simulink model "drone_nao_linear_V3_MF_LQR"  (R2015a)
settings: Solver=ode45  StartTime=0.0  StopTime=30  FixedStep=.001  RelTol=1e-3
values from neighbouring files (symbols this model uses):
  Cx = 1.33    [projeto_Drone_LQR_pratico.m]
  Cy = 1.95    [projeto_Drone_LQR_pratico.m]
  d_fi = 1.35    [projeto_Drone_LQR_pratico.m]
  d_teta = 0.99    [projeto_Drone_LQR_pratico.m]
  Fi_max = 0.4171/2    (= 0.20855)    [projeto_Drone_LQR_pratico.m]
  g = 0.165/(pi/180)    (= 9.45380361966)    [projeto_Drone_LQR_pratico.m]
  K_psi_p = 1    [projeto_Drone_LQR_pratico.m]
  K_z_p = 1    [projeto_Drone_LQR_pratico.m]
  Kipsi = -Ka_psi(1,3)    [projeto_Drone_LQR_pratico.m]
  Kix = -Ka_x(1,5)    [projeto_Drone_LQR_pratico.m]
  Kiy = -Ka_y(1,5)    [projeto_Drone_LQR_pratico.m]
  Kiz = -Ka_z(1,3)    [projeto_Drone_LQR_pratico.m]
  Kpsi = -Ka_psi(1,1:2)    [projeto_Drone_LQR_pratico.m]
  Kx = -Ka_x(1,1:4)    [projeto_Drone_LQR_pratico.m]
  Ky = -Ka_y(1,1:4)    [projeto_Drone_LQR_pratico.m]
  Kz = -Ka_z(1,1:2)    [projeto_Drone_LQR_pratico.m]
  omega_fi = 14.43    [projeto_Drone_LQR_pratico.m]
  omega_teta = 13.14    [projeto_Drone_LQR_pratico.m]
  Psi_p_max = 92.75*(pi/180)    (= 1.61879288122)    [projeto_Drone_LQR_pratico.m]
  T = 5    [projeto_Drone_LQR_pratico.m]
  Tau_psi_p = 0.51    [projeto_Drone_LQR_pratico.m]
  Tau_z_p = 0.88    [projeto_Drone_LQR_pratico.m]
  Teta_max = 0.4184/2    (= 0.2092)    [projeto_Drone_LQR_pratico.m]
  z_p_max = 1.35    [projeto_Drone_LQR_pratico.m]
libraries: simulink_extras x3
settings Model: Creator=Humberto  LastModifiedBy=Humberto

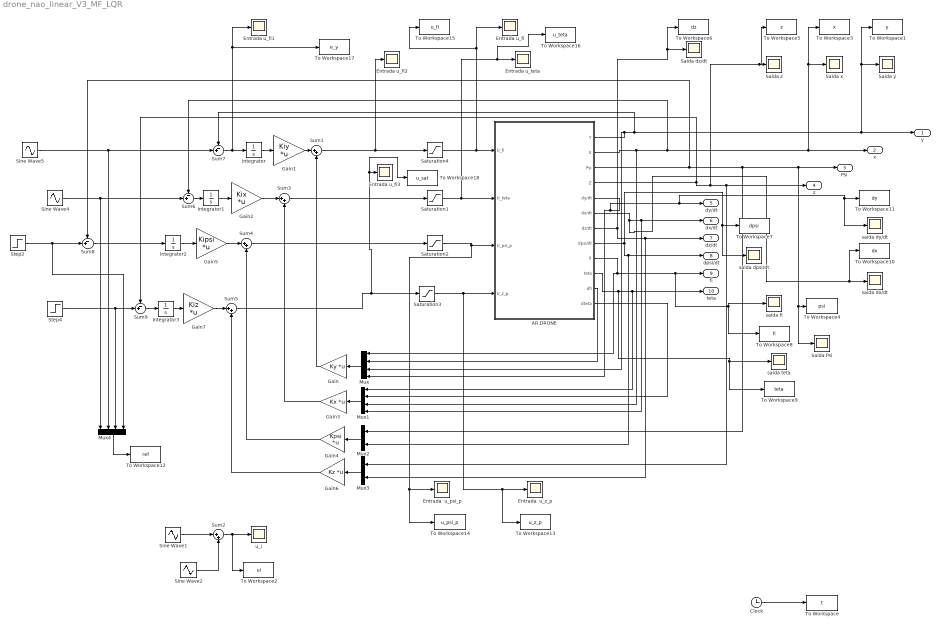
== system drone_nao_linear_V3_MF_LQR ==
  AR.DRONE : Subsystem
      mask Display: color('blue');port_label('output',1,'x')
  Clock : Clock
  Entrada  u_psi_p : Scope
      settings: SaveName=ScopeData17
  Entrada  u_z_p : Scope
      settings: SaveName=ScopeData16
  Entrada u_fi{,1..3} (4 alike) : Scope
      Entrada u_fi settings: SaveName=ScopeData14
      Entrada u_fi1 settings: SaveName=ScopeData22
      Entrada u_fi2 settings: SaveName=ScopeData23
      Entrada u_fi3 settings: SaveName=ScopeData24
  Entrada u_teta : Scope
      settings: SaveName=ScopeData15
  Gain : Gain  Gain=Ky  Multiplication=Matrix(K*u)
  Gain1 : Gain  Gain=Kiy  Multiplication=Matrix(K*u)
  Gain2 : Gain  Gain=Kix  Multiplication=Matrix(K*u)
  Gain3 : Gain  Gain=Kx  Multiplication=Matrix(K*u)
  Gain4 : Gain  Gain=Kpsi  Multiplication=Matrix(K*u)
  Gain5 : Gain  Gain=Kipsi  Multiplication=Matrix(K*u)
  Gain6 : Gain  Gain=Kz  Multiplication=Matrix(K*u)
  Gain7 : Gain  Gain=Kiz  Multiplication=Matrix(K*u)
  Integrator{,1..3} (4 alike) : Integrator
  Mux : Mux
  Mux1 : Mux
  Mux2 : Mux  Inputs=2
  Mux3 : Mux  Inputs=2
  Mux4 : Mux
  Saida Psi : Scope
      settings: SaveName=ScopeData2
  Saida dz/dt : Scope
      settings: SaveName=ScopeData19
  Saida x : Scope
  Saida y : Scope
  Saida z : Scope
      settings: SaveName=ScopeData3
  Saturation{1..4} (4 alike) : Saturate  UpperLimit=1  LowerLimit=-1
  Sine Wave1 : Sin  Amplitude=0.5  Frequency=2*pi/T  SampleTime=0
  Sine Wave2 : Sin  Amplitude=0.3  Frequency=2*pi/(0.2*T)  SampleTime=0
  Sine Wave4 : Sin  Frequency=0.8  SampleTime=0
  Sine Wave5 : Sin  Frequency=0.8  Phase=pi/2  SampleTime=0
  Step2 : Step  Time=0  After=0  SampleTime=0
  Step4 : Step  Time=0  After=1.2  SampleTime=0
  Sum{1..5} (5 alike) : Sum  Inputs=|++
  Sum{6..9} (4 alike) : Sum  Inputs=-+|
  To Workspace : ToWorkspace  VariableName=t  SampleTime=-1
  To Workspace1 : ToWorkspace  VariableName=y  SampleTime=-1
  To Workspace10 : ToWorkspace  VariableName=dx  SampleTime=-1
  To Workspace11 : ToWorkspace  VariableName=dy  SampleTime=-1
  To Workspace12 : ToWorkspace  VariableName=ref  SampleTime=-1
  To Workspace13 : ToWorkspace  VariableName=u_z_p  SampleTime=-1
  To Workspace14 : ToWorkspace  VariableName=u_psi_p  SampleTime=-1
  To Workspace15 : ToWorkspace  VariableName=u_fi  SampleTime=-1
  To Workspace16 : ToWorkspace  VariableName=u_teta  SampleTime=-1
  To Workspace17 : ToWorkspace  VariableName=e_y  SampleTime=-1
  To Workspace18 : ToWorkspace  VariableName=u_sat  SampleTime=-1
  To Workspace2 : ToWorkspace  VariableName=ui  SampleTime=-1
  To Workspace3 : ToWorkspace  VariableName=x  SampleTime=-1
  To Workspace4 : ToWorkspace  VariableName=psi  SampleTime=-1
  To Workspace5 : ToWorkspace  VariableName=z  SampleTime=-1
  To Workspace6 : ToWorkspace  VariableName=dz  SampleTime=-1
  To Workspace7 : ToWorkspace  VariableName=dpsi  SampleTime=-1
  To Workspace8 : ToWorkspace  VariableName=fi  SampleTime=-1
  To Workspace9 : ToWorkspace  VariableName=teta  SampleTime=-1
  saida dpsi/dt : Scope
      settings: SaveName=ScopeData13
  saida dx/dt : Scope
      settings: SaveName=ScopeData20
  saida dy/dt : Scope
      settings: SaveName=ScopeData21
  saida fi : Scope
      settings: SaveName=ScopeData10
  saida teta : Scope
      settings: SaveName=ScopeData18
  u_i : Scope
      settings: YMin=-1  YMax=1  SaveName=ScopeData8
  y : Outport
  x : Outport  Port=2
  Psi : Outport  Port=3
  z : Outport  Port=4
  dy/dt : Outport  Port=5
  dx/dt : Outport  Port=6
  dz/dt : Outport  Port=7
  dpsi/dt : Outport  Port=8
  fi : Outport  Port=9
  teta : Outport  Port=10
  wires:
  AR.DRONE/10(teta) -> To Workspace9/1, saida teta/1, Mux1/1, teta/1
  AR.DRONE/5(dy/dt) -> saida dy/dt/1, To Workspace11/1, dy/dt/1, Mux/4
  AR.DRONE/7(dz/dt) -> Mux3/2, dz/dt/1, To Workspace6/1, Saida dz/dt/1
  AR.DRONE/9(fi) -> Mux/1, To Workspace8/1, saida fi/1, fi/1
  Saturation4/1 -> AR.DRONE/1(U_fi), Entrada u_fi/1, To Workspace15/1
  Saturation3/1 -> AR.DRONE/4(U_z_p), To Workspace13/1, Entrada  u_z_p/1
  Saturation1/1 -> AR.DRONE/2(U_teta), To Workspace16/1, Entrada u_teta/1
  Saturation2/1 -> To Workspace14/1, Entrada  u_psi_p/1, AR.DRONE/3(U_psi_p)
  Clock/1 -> To Workspace/1
  AR.DRONE/4(Z) -> To Workspace5/1, Saida z/1, Mux3/1, z/1, Sum9/1
  AR.DRONE/3(Psi) -> Mux2/1, Saida Psi/1, To Workspace4/1, Psi/1, Sum8/1
  AR.DRONE/8(dpsi/dt) -> Mux2/2, dpsi/dt/1, To Workspace7/1, saida dpsi/dt/1
  Sine Wave1/1 -> Sum2/1
  Sine Wave2/1 -> Sum2/2
  Sum2/1 -> To Workspace2/1, u_i/1
  Sum4/1 -> Saturation2/1
  Sum5/1 -> To Workspace18/1, Entrada u_fi3/1, Saturation3/1
  Sum1/1 -> Entrada u_fi2/1, Saturation4/1
  Mux/1 -> Gain/1
  Gain/1 -> Sum1/2
  Integrator/1 -> Gain1/1
  Sine Wave5/1 -> Sum7/2, Mux4/2
  Sum7/1 -> To Workspace17/1, Entrada u_fi1/1, Integrator/1
  Gain1/1 -> Sum1/1
  AR.DRONE/1(Y) -> Sum7/1, y/1, Saida y/1, To Workspace1/1, Mux/3
  AR.DRONE/2(X) -> Sum6/1, Saida x/1, To Workspace3/1, x/1, Mux1/3
  AR.DRONE/6(dx/dt) -> saida dx/dt/1, To Workspace10/1, Mux1/4, dx/dt/1
  Mux1/1 -> Gain3/1
  Gain2/1 -> Sum3/1
  Integrator1/1 -> Gain2/1
  Sum6/1 -> Integrator1/1
  Sine Wave4/1 -> Sum6/2, Mux4/1
  Gain3/1 -> Sum3/2
  Sum3/1 -> Saturation1/1
  Mux2/1 -> Gain4/1
  Gain4/1 -> Sum4/2
  Gain5/1 -> Sum4/1
  Step2/1 -> Mux4/4, Sum8/2
  Sum8/1 -> Integrator2/1
  Integrator2/1 -> Gain5/1
  Gain6/1 -> Sum5/2
  Gain7/1 -> Sum5/1
  Sum9/1 -> Integrator3/1
  Step4/1 -> Sum9/2, Mux4/3
  Integrator3/1 -> Gain7/1
  Mux3/1 -> Gain6/1
  AR.DRONE/12(dteta) -> Mux1/2
  AR.DRONE/11(dfi) -> Mux/2
  Mux4/1 -> To Workspace12/1

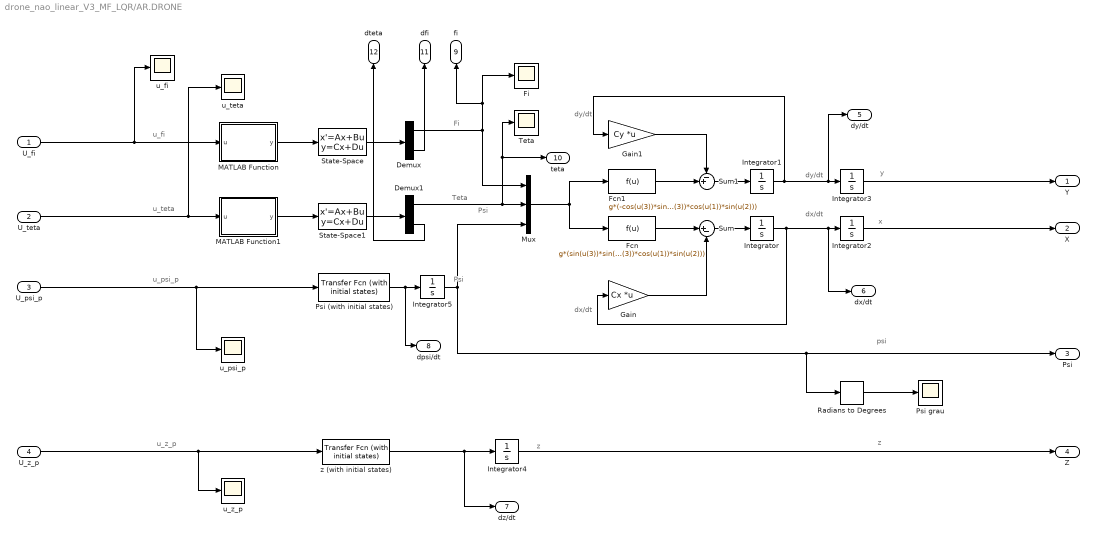
== system drone_nao_linear_V3_MF_LQR/AR.DRONE ==
  note: z
  note: psi
  note: Psi
  note: Teta
  note: Fi
  note: u_fi
  note: Psi
  note: y
  note: dx/dt
  note: dy/dt
  note: x
  note: dx/dt
  note: dy/dt
  note: u_teta
  note: u_psi_p
  note: u_z_p
  note: z
  U_fi : Inport
  U_teta : Inport  Port=2
  U_psi_p : Inport  Port=3
  U_z_p : Inport  Port=4
  Demux : Demux  Outputs=2
  Demux1 : Demux  Outputs=2
  Fcn : Fcn  Expr=g*(sin(u(3))*sin(u(1))+cos(u(3))*cos(u(1))*sin(u(2)))
  Fcn1 : Fcn  Expr=g*(-cos(u(3))*sin(u(1))+sin(u(3))*cos(u(1))*sin(u(2)))
  Fi : Scope
      settings: SaveName=ScopeData5
  Gain : Gain  Gain=Cx  Multiplication=Matrix(K*u)
  Gain1 : Gain  Gain=Cy  Multiplication=Matrix(K*u)
  Integrator{,1..5} (6 alike) : Integrator
  MATLAB Function : MATLAB Function  TreatAsAtomicUnit=on
  MATLAB Function1 : MATLAB Function  TreatAsAtomicUnit=on
  Mux : Mux  Inputs=3
  Psi (with initial states) : simulink_extras/Additional Linear/Transfer Fcn (with initial states)  N=K_psi_p*Psi_p_max  D=[Tau_psi_p 1]  X0=[0]
  Psi grau : Scope
      settings: SaveName=ScopeData4
  Radians to Degrees : simulink_extras/Transformations/Radians to Degrees
  State-Space : StateSpace  A=[0 1;-omega_fi^2 -2*d_fi*omega_fi]  B=[0 Fi_max*(omega_fi^2)]'  C=eye(2)  D=[0 0]'  X0=0
  State-Space1 : StateSpace  A=[0 1;-omega_teta^2 -2*d_teta*omega_teta]  B=[0 Teta_max*(omega_teta^2)]'  C=eye(2)  D=[0 0]'  X0=0
  Sum : Sum  Inputs=|+-
  Sum1 : Sum  Inputs=-+|
  Teta : Scope
      settings: SaveName=ScopeData7
  u_fi : Scope
      settings: SaveName=ScopeData6
  u_psi_p : Scope
      settings: SaveName=ScopeData11
  u_teta : Scope
      settings: SaveName=ScopeData9
  u_z_p : Scope
      settings: SaveName=ScopeData12
  z (with initial states) : simulink_extras/Additional Linear/Transfer Fcn (with initial states)  N=K_z_p*z_p_max  D=[Tau_z_p 1]  X0=[0]
  Y : Outport
  X : Outport  Port=2
  Psi : Outport  Port=3
  Z : Outport  Port=4
  dy/dt : Outport  Port=5
  dx/dt : Outport  Port=6
  dz/dt : Outport  Port=7
  dpsi/dt : Outport  Port=8
  fi : Outport  Port=9
  teta : Outport  Port=10
  dfi : Outport  Port=11
  dteta : Outport  Port=12
  wires:
  Integrator1/1 -> dy/dt/1, Integrator3/1, Gain1/1
  Sum/1 -> Integrator/1
  Fcn/1 -> Sum/1
  Integrator/1 -> dx/dt/1, Integrator2/1, Gain/1
  Gain/1 -> Sum/2
  z (with initial states)/1 -> dz/dt/1, Integrator4/1
  Radians to Degrees/1 -> Psi grau/1
  U_z_p/1 -> z (with initial states)/1, u_z_p/1
  U_fi/1 -> u_fi/1, MATLAB Function/1(u)
  Psi (with initial states)/1 -> dpsi/dt/1, Integrator5/1
  U_psi_p/1 -> u_psi_p/1, Psi (with initial states)/1
  U_teta/1 -> u_teta/1, MATLAB Function1/1(u)
  Gain1/1 -> Sum1/1
  Sum1/1 -> Integrator1/1
  Fcn1/1 -> Sum1/2
  Demux/1 -> Mux/1, Fi/1, fi/1
  MATLAB Function/1(y) -> State-Space/1
  MATLAB Function1/1(y) -> State-Space1/1
  Integrator3/1 -> Y/1
  Mux/1 -> Fcn1/1, Fcn/1
  Demux1/1 -> teta/1, Teta/1, Mux/2
  Integrator4/1 -> Z/1
  Integrator5/1 -> Mux/3, Radians to Degrees/1, Psi/1
  Integrator2/1 -> X/1
  State-Space/1 -> Demux/1
  Demux/2 -> dfi/1
  State-Space1/1 -> Demux1/1
  Demux1/2 -> dteta/1

== matlab function drone_nao_linear_V3_MF_LQR/AR.DRONE/MATLAB Function1 ==
  data: u input; y output
function y = myfcn2(u)

K_teta_min = 1;
K_teta_max = 2;

if abs(u)>=0.5
    u=K_teta_min*u;
else
    u=K_teta_max*u;
end

y = u;

== matlab function drone_nao_linear_V3_MF_LQR/AR.DRONE/MATLAB Function ==
  data: u input; y output
function y = myfcn1(u)
K_fi_min = 1;
K_fi_max = 2;
if abs(u)>=0.5
    u=K_fi_min*u;
else
    u=K_fi_max*u;
end

y = u;
